simulink model "Warning_Detection"  (R2024b)
settings: Solver=VariableStepAuto  StartTime=0.0  StopTime=30  RelTol=1e-3
libraries: simulink x5
settings Model: Creator=Michele  LastModifiedBy=Michele
settings ConfigComp: CovMetricSettings=dcmwe

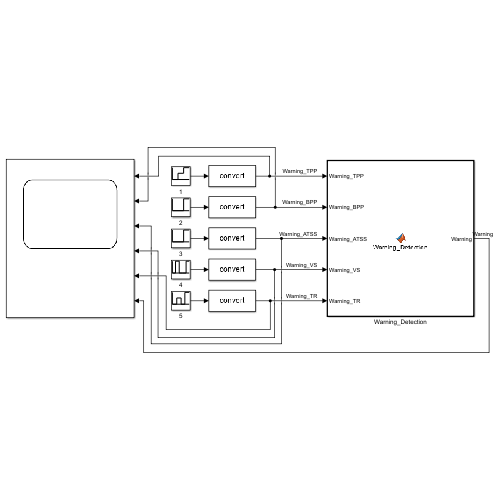
[thumbnail: Simulink's stored preview of the top-level diagram]
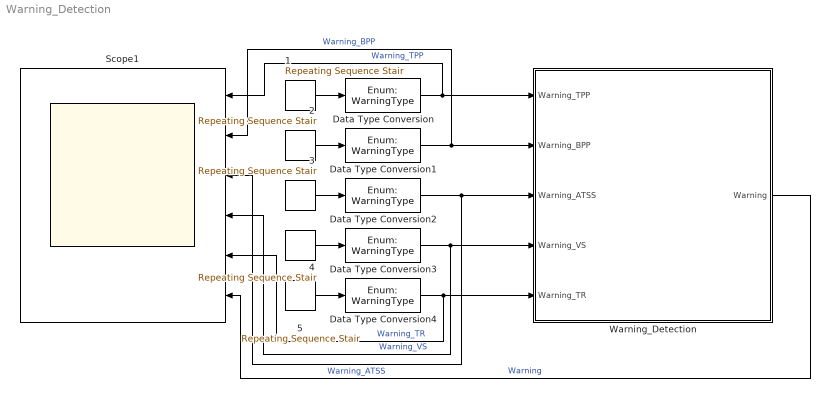
== system Warning_Detection ==
  1 : simulink/Sources/Repeating Sequence Stair  OutValues=[0 1 2].'  tsamp=2  OutMin=[]  OutMax=[]  OutDataTypeStr=uint8  OutputDataTypeScalingMode=uint8  OutDataType=Enum: TransmissionState  ConRadixGroup=Best Precision: Vector-wise  OutScaling=[]
  2 : simulink/Sources/Repeating Sequence Stair  OutValues=[0 0 2].'  tsamp=2  OutMin=[]  OutMax=[]  OutDataTypeStr=uint8  OutputDataTypeScalingMode=uint8  OutDataType=Enum: TransmissionState  ConRadixGroup=Best Precision: Vector-wise  OutScaling=[]
  3 : simulink/Sources/Repeating Sequence Stair  OutValues=[0 0 2].'  tsamp=4  OutMin=[]  OutMax=[]  OutDataTypeStr=uint8  OutputDataTypeScalingMode=uint8  OutDataType=Enum: TransmissionState  ConRadixGroup=Best Precision: Vector-wise  OutScaling=[]
  4 : simulink/Sources/Repeating Sequence Stair  OutValues=[0 1 0 0 1].'  tsamp=1  OutMin=[]  OutMax=[]  OutDataTypeStr=uint8  OutputDataTypeScalingMode=uint8  OutDataType=Enum: TransmissionState  ConRadixGroup=Best Precision: Vector-wise  OutScaling=[]
  5 : simulink/Sources/Repeating Sequence Stair  OutValues=[0 1 0 2].'  tsamp=2  OutMin=[]  OutMax=[]  OutDataTypeStr=uint8  OutputDataTypeScalingMode=uint8  OutDataType=Enum: TransmissionState  ConRadixGroup=Best Precision: Vector-wise  OutScaling=[]
  Data Type Conversion{,1..4} (5 alike) : DataTypeConversion  OutDataTypeStr=Enum: WarningType  SaturateOnIntegerOverflow=off  RndMeth=Floor
  Scope1 : Scope  NumInputPorts=6
  Warning_Detection : MATLAB Function  TreatAsAtomicUnit=on
  wires:
  1/1 -> Data Type Conversion/1
  Data Type Conversion3/1 -> Scope1/4, Warning_Detection/4(Warning_VS)  "Warning_VS"
  Data Type Conversion4/1 -> Scope1/5, Warning_Detection/5(Warning_TR)  "Warning_TR"
  Warning_Detection/1(Warning) -> Scope1/6  "Warning"
  Data Type Conversion2/1 -> Scope1/3, Warning_Detection/3(Warning_ATSS)  "Warning_ATSS"
  Data Type Conversion1/1 -> Warning_Detection/2(Warning_BPP), Scope1/2  "Warning_BPP"
  Data Type Conversion/1 -> Scope1/1, Warning_Detection/1(Warning_TPP)  "Warning_TPP"
  2/1 -> Data Type Conversion1/1
  3/1 -> Data Type Conversion2/1
  4/1 -> Data Type Conversion3/1
  5/1 -> Data Type Conversion4/1

== matlab function Warning_Detection/Warning_Detection ==
  data: Warning_TPP input Enum: WarningType; Warning output Enum: WarningType; Warning_BPP input Enum: WarningType; Warning_ATSS input Enum: WarningType; Warning_VS input Enum: WarningType; Warning_TR input Enum: WarningType
function Warning = Warning_Detection(Warning_TPP,Warning_BPP,Warning_ATSS,Warning_VS,Warning_TR)

Warning =  WarningType(0);

Warning_set = [Warning_TPP,Warning_BPP,Warning_ATSS,Warning_VS,Warning_TR];

if any(Warning_set ==  WarningType(1))

    Warning =  WarningType(1);

     if any(Warning_set == WarningType(2))
    
        Warning = WarningType(2);
    
     end

elseif any(Warning_set == WarningType(2))

    Warning = WarningType(2);

end
